simulink model "lab02_3"  (Simulink 10.3)
settings: Solver=VariableStepAuto  StartTime=0.0  StopTime=10  RelTol=1e-3
values from neighbouring files (symbols this model uses):
  Denth = [1 1.28221624265 36.6770172992 23.5454339835 -528.584013296]    [lab03.mat]    (also in lab04.mat; lab05.mat; lab06.mat; lab07.mat)
  Denx = [1 1.28221624265 36.6770172992 23.5454339835 -528.584013296]    [lab03.mat]    (also in lab04.mat; lab05.mat; lab06.mat; lab07.mat)
  k_a = 2546    [lab02.mat]    (also in lab03.mat; lab04.mat; lab05.mat; lab06.mat)
  k_f = 0.0013    [lab02.mat]    (also in lab03.mat; lab04.mat; lab05.mat; lab06.mat)
  k_s = 32    [lab02.mat]    (also in lab03.mat; lab04.mat; lab05.mat; lab06.mat)
  k_x = 50200    [lab02.mat]    (also in lab03.mat; lab04.mat; lab05.mat; lab06.mat)
  Numth = [0 0 -7.64415309154 -7.25165028128 227.008182718]    [lab03.mat]    (also in lab04.mat; lab05.mat; lab06.mat; lab07.mat)
  Numx = [0 0 6.73132472896 2.24532116671 3.20735046038]    [lab03.mat]    (also in lab04.mat; lab05.mat; lab06.mat; lab07.mat)
settings Model: Creator=kisdev  LastModifiedBy=kisdev
settings SolverCC: AlgebraicLoopSolver=Auto
settings DataIOCC: SaveFormat=Dataset  SignalLoggingSaveFormat=Dataset  ReturnWorkspaceOutputs=on
settings OptimizationCC: ExpressionDepthLimit=128  LifeSpan=auto
settings DebuggingCC: UnderspecifiedInitializationDetection=Simplified  MergeDetectMultiDrivingBlocksExec=error  FcnCallInpInsideContextMsg=error  StateNameClashWarn=none  SFUnexpectedBacktrackingDiag=error  SFNoUnconditionalDefaultTransitionDiag=error  SFExecutionAtInitializationDiag=warning  SFMachineParentedDataDiag=error  ArithmeticOperatorsInVariantConditions=error
settings HardwareCC: ProdBitPerPointer=64  ProdBitPerSizeT=64  ProdBitPerPtrDiffT=64  ProdLargestAtomicFloat=Float  ProdIntDivRoundTo=Zero  ProdEndianess=LittleEndian  ProdWordSize=64  ProdHWDeviceType=Intel->x86-64 (Windows64)
settings ModelReferenceCC: PropagateSignalLabelsOutOfModel=on
settings SFSimCC: SimUseLocalCustomCode=on  CustomCodeUndefinedFunction=FilterOut
settings RTWCC: RTWUseLocalCustomCode=on
settings CodeAppCC: StateflowObjectComments=off
settings GRTTargetCC: TargetLangStandard=C99 (ISO)  CombineOutputUpdateFcns=on  GRTInterface=off
settings ConfigComp: CovMetricSettings=dwe  CovSaveCumulativeToWorkspaceVar=off  CovSaveSingleToWorkspaceVar=off  CovExternalEMLEnable=on

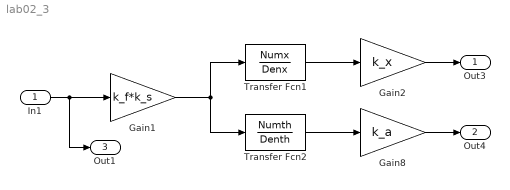
== system lab02_3 ==
  In1 : Inport
  Gain1 : Gain  Gain=k_f*k_s
  Gain2 : Gain  Gain=k_x
  Gain8 : Gain  Gain=k_a
  Transfer Fcn1 : TransferFcn  Numerator=Numx  Denominator=Denx
  Transfer Fcn2 : TransferFcn  Numerator=Numth  Denominator=Denth
  Out3 : Outport  SignalName=x
  Out4 : Outport  Port=2  SignalName=theta
  Out1 : Outport  Port=3  SignalName=in
  wires:
  In1/1 -> Out1/1, Gain1/1
  Gain1/1 -> Transfer Fcn2/1, Transfer Fcn1/1
  Gain2/1 -> Out3/1
  Transfer Fcn1/1 -> Gain2/1
  Gain8/1 -> Out4/1
  Transfer Fcn2/1 -> Gain8/1
